simulink model "x12_agv"  (R2025a)
settings: Solver=VariableStepAuto  StartTime=0.0  StopTime=30  RelTol=1e-3
undefined symbols (not defined in the file): Ad, Bd, d_sel, K, kc_pos, kc_vel, p, ref_1, ref_10, ref_11, ref_12, ref_2, ref_3, ref_4, ref_5, ref_6, ref_7, ref_8, ref_9, Ts, x0, x0_1, x0_10, x0_11, x0_12, x0_2, x0_3, x0_4, x0_5, x0_6, x0_7, x0_8, x0_9
(part 2 of 2)

== system x12_agv/agv_init ==
  ref_in : Inport
  p_in : Inport  Port=2
  d_sel_in : Inport  Port=3
  Constant : Constant
  DelaySel : MultiPortSwitch  DataPortOrder=Specify indices  DiagnosticForDefault=None  SaturateOnIntegerOverflow=off  InputSameDT=off
  Gain_k : Gain  Gain=K  Multiplication=Matrix(K*u)
  Gain_neg1 : Gain  Gain=-1  Multiplication=Matrix(K*u)
  Produc_lt : Product
  Product_g : Product
  Relational Operator : RelationalOperator  OutDataTypeStr=boolean  RndMeth=Simplest  InputSameDT=off
  Sum-e : Sum  Inputs=|+-
  plant : DiscreteStateSpace  A=Ad  B=Bd  C=eye(4)  D=zeros(4,2)  InitialCondition=x0  SampleTime=Ts
  sum2 : Sum  Inputs=|++
  sum3 : Sum  Inputs=|++
  ud_u1 : UnitDelay  InitialCondition=[0;0]  SampleTime=Ts  HasFrameUpgradeWarning=on
  ud_u2 : UnitDelay  InitialCondition=[0;0]  SampleTime=Ts  HasFrameUpgradeWarning=on
  ud_u3 : UnitDelay  InitialCondition=[0;0]  SampleTime=Ts  HasFrameUpgradeWarning=on
  ud_ua_prev : UnitDelay  InitialCondition=[0;0]  SampleTime=Ts  HasFrameUpgradeWarning=on
  uniformrandom : UniformRandomNumber  Minimum=0  SampleTime=Ts
  x_out : Outport
  ua_out : Outport  Port=2
  gamma_out : Outport  Port=3
  wires:
  ud_u1/1 -> ud_u2/1, DelaySel/2
  Relational Operator/1 -> gamma_out/1, Product_g/2, Gain_neg1/1
  ud_u3/1 -> DelaySel/4
  plant/1 -> Sum-e/1, x_out/1
  Produc_lt/1 -> sum3/2
  sum2/1 -> Produc_lt/1
  ud_ua_prev/1 -> Produc_lt/2
  Constant/1 -> sum2/2
  Gain_neg1/1 -> sum2/1
  DelaySel/1 -> Product_g/1
  Product_g/1 -> sum3/1
  Gain_k/1 -> ud_u1/1
  ud_u2/1 -> ud_u3/1, DelaySel/3
  Sum-e/1 -> Gain_k/1
  sum3/1 -> ud_ua_prev/1, plant/1, ua_out/1
  uniformrandom/1 -> Relational Operator/1
  ref_in/1 -> Sum-e/2
  p_in/1 -> Relational Operator/2
  d_sel_in/1 -> DelaySel/1

== matlab function x12_agv/Ucoop_8/MATLAB Function ==
  data: xi input; u_coop output; xj1 input; xj2 input; xj3 input; kc_pos input; kc_vel input; u_rep output
function [u_coop, u_rep] = fcn(xi, xj1, xj2, xj3, kc_pos, kc_vel)
% xi, xj1, xj2, xj3: [4x1] = [px; py; vx; vy]

% ----- fixed repulsion params -----
d_safe = 0.45;
k_rep  = 2.4;

% ----- cooperative term (2-neighbor) -----
pi  = xi(1:2);
vi  = xi(3:4);

pj1 = xj1(1:2); vj1 = xj1(3:4);
pj2 = xj2(1:2); vj2 = xj2(3:4);
pj3 = xj3(1:2); % repulsion-only neighbor

e_pos = (pi - pj1) + (pi - pj2);
e_vel = (vi - vj1) + (vi - vj2);

u_coop_base = -kc_pos * e_pos - kc_vel * e_vel;

% ----- repulsion term (3 constraints) -----
eps_d = 1e-6;
u_rep = [0; 0];

% j1
dp = pi - pj1;
d = norm(dp);
if d < d_safe
    u_rep = u_rep + k_rep * (d_safe - d) * (dp / (d + eps_d));
end

% j2
dp = pi - pj2;
d = norm(dp);
if d < d_safe
    u_rep = u_rep + k_rep * (d_safe - d) * (dp / (d + eps_d));
end

% j3
dp = pi - pj3;
d = norm(dp);
if d < d_safe
    u_rep = u_rep + k_rep * (d_safe - d) * (dp / (d + eps_d));
end

% output-1 keeps original channel name u_coop, now includes repulsion
u_coop = u_coop_base + u_rep;
end

== matlab function x12_agv/Ucoop_9/MATLAB Function ==
  data: xi input; u_coop output; xj1 input; xj2 input; xj3 input; kc_pos input; kc_vel input; u_rep output
function [u_coop, u_rep] = fcn(xi, xj1, xj2, xj3, kc_pos, kc_vel)
% xi, xj1, xj2, xj3: [4x1] = [px; py; vx; vy]

% ----- fixed repulsion params -----
d_safe = 0.45;
k_rep  = 2.4;

% ----- cooperative term (2-neighbor) -----
pi  = xi(1:2);
vi  = xi(3:4);

pj1 = xj1(1:2); vj1 = xj1(3:4);
pj2 = xj2(1:2); vj2 = xj2(3:4);
pj3 = xj3(1:2); % repulsion-only neighbor

e_pos = (pi - pj1) + (pi - pj2);
e_vel = (vi - vj1) + (vi - vj2);

u_coop_base = -kc_pos * e_pos - kc_vel * e_vel;

% ----- repulsion term (3 constraints) -----
eps_d = 1e-6;
u_rep = [0; 0];

% j1
dp = pi - pj1;
d = norm(dp);
if d < d_safe
    u_rep = u_rep + k_rep * (d_safe - d) * (dp / (d + eps_d));
end

% j2
dp = pi - pj2;
d = norm(dp);
if d < d_safe
    u_rep = u_rep + k_rep * (d_safe - d) * (dp / (d + eps_d));
end

% j3
dp = pi - pj3;
d = norm(dp);
if d < d_safe
    u_rep = u_rep + k_rep * (d_safe - d) * (dp / (d + eps_d));
end

% output-1 keeps original channel name u_coop, now includes repulsion
u_coop = u_coop_base + u_rep;
end

== matlab function x12_agv/Ucoop_10/MATLAB Function ==
  data: xi input; u_coop output; xj1 input; xj2 input; xj3 input; kc_pos input; kc_vel input; u_rep output
function [u_coop, u_rep] = fcn(xi, xj1, xj2, xj3, kc_pos, kc_vel)
% xi, xj1, xj2, xj3: [4x1] = [px; py; vx; vy]

% ----- fixed repulsion params -----
d_safe = 0.45;
k_rep  = 2.4;

% ----- cooperative term (2-neighbor) -----
pi  = xi(1:2);
vi  = xi(3:4);

pj1 = xj1(1:2); vj1 = xj1(3:4);
pj2 = xj2(1:2); vj2 = xj2(3:4);
pj3 = xj3(1:2); % repulsion-only neighbor

e_pos = (pi - pj1) + (pi - pj2);
e_vel = (vi - vj1) + (vi - vj2);

u_coop_base = -kc_pos * e_pos - kc_vel * e_vel;

% ----- repulsion term (3 constraints) -----
eps_d = 1e-6;
u_rep = [0; 0];

% j1
dp = pi - pj1;
d = norm(dp);
if d < d_safe
    u_rep = u_rep + k_rep * (d_safe - d) * (dp / (d + eps_d));
end

% j2
dp = pi - pj2;
d = norm(dp);
if d < d_safe
    u_rep = u_rep + k_rep * (d_safe - d) * (dp / (d + eps_d));
end

% j3
dp = pi - pj3;
d = norm(dp);
if d < d_safe
    u_rep = u_rep + k_rep * (d_safe - d) * (dp / (d + eps_d));
end

% output-1 keeps original channel name u_coop, now includes repulsion
u_coop = u_coop_base + u_rep;
end

== matlab function x12_agv/Ucoop_11/MATLAB Function ==
  data: xi input; u_coop output; xj1 input; xj2 input; xj3 input; kc_pos input; kc_vel input; u_rep output
function [u_coop, u_rep] = fcn(xi, xj1, xj2, xj3, kc_pos, kc_vel)
% xi, xj1, xj2, xj3: [4x1] = [px; py; vx; vy]

% ----- fixed repulsion params -----
d_safe = 0.45;
k_rep  = 2.4;

% ----- cooperative term (2-neighbor) -----
pi  = xi(1:2);
vi  = xi(3:4);

pj1 = xj1(1:2); vj1 = xj1(3:4);
pj2 = xj2(1:2); vj2 = xj2(3:4);
pj3 = xj3(1:2); % repulsion-only neighbor

e_pos = (pi - pj1) + (pi - pj2);
e_vel = (vi - vj1) + (vi - vj2);

u_coop_base = -kc_pos * e_pos - kc_vel * e_vel;

% ----- repulsion term (3 constraints) -----
eps_d = 1e-6;
u_rep = [0; 0];

% j1
dp = pi - pj1;
d = norm(dp);
if d < d_safe
    u_rep = u_rep + k_rep * (d_safe - d) * (dp / (d + eps_d));
end

% j2
dp = pi - pj2;
d = norm(dp);
if d < d_safe
    u_rep = u_rep + k_rep * (d_safe - d) * (dp / (d + eps_d));
end

% j3
dp = pi - pj3;
d = norm(dp);
if d < d_safe
    u_rep = u_rep + k_rep * (d_safe - d) * (dp / (d + eps_d));
end

% output-1 keeps original channel name u_coop, now includes repulsion
u_coop = u_coop_base + u_rep;
end

== matlab function x12_agv/Ucoop_3/MATLAB Function ==
  data: xi input; u_coop output; xj1 input; xj2 input; xj3 input; kc_pos input; kc_vel input; u_rep output
function [u_coop, u_rep] = fcn(xi, xj1, xj2, xj3, kc_pos, kc_vel)
% xi, xj1, xj2, xj3: [4x1] = [px; py; vx; vy]

% ----- fixed repulsion params -----
d_safe = 0.45;
k_rep  = 2.4;

% ----- cooperative term (2-neighbor) -----
pi  = xi(1:2);
vi  = xi(3:4);

pj1 = xj1(1:2); vj1 = xj1(3:4);
pj2 = xj2(1:2); vj2 = xj2(3:4);
pj3 = xj3(1:2); % repulsion-only neighbor

e_pos = (pi - pj1) + (pi - pj2);
e_vel = (vi - vj1) + (vi - vj2);

u_coop_base = -kc_pos * e_pos - kc_vel * e_vel;

% ----- repulsion term (3 constraints) -----
eps_d = 1e-6;
u_rep = [0; 0];

% j1
dp = pi - pj1;
d = norm(dp);
if d < d_safe
    u_rep = u_rep + k_rep * (d_safe - d) * (dp / (d + eps_d));
end

% j2
dp = pi - pj2;
d = norm(dp);
if d < d_safe
    u_rep = u_rep + k_rep * (d_safe - d) * (dp / (d + eps_d));
end

% j3
dp = pi - pj3;
d = norm(dp);
if d < d_safe
    u_rep = u_rep + k_rep * (d_safe - d) * (dp / (d + eps_d));
end

% output-1 keeps original channel name u_coop, now includes repulsion
u_coop = u_coop_base + u_rep;
end

== matlab function x12_agv/Ucoop_12/MATLAB Function ==
  data: xi input; u_coop output; xj1 input; xj2 input; xj3 input; kc_pos input; kc_vel input; u_rep output
function [u_coop, u_rep] = fcn(xi, xj1, xj2, xj3, kc_pos, kc_vel)
% xi, xj1, xj2, xj3: [4x1] = [px; py; vx; vy]

% ----- fixed repulsion params -----
d_safe = 0.45;
k_rep  = 2.4;

% ----- cooperative term (2-neighbor) -----
pi  = xi(1:2);
vi  = xi(3:4);

pj1 = xj1(1:2); vj1 = xj1(3:4);
pj2 = xj2(1:2); vj2 = xj2(3:4);
pj3 = xj3(1:2); % repulsion-only neighbor

e_pos = (pi - pj1) + (pi - pj2);
e_vel = (vi - vj1) + (vi - vj2);

u_coop_base = -kc_pos * e_pos - kc_vel * e_vel;

% ----- repulsion term (3 constraints) -----
eps_d = 1e-6;
u_rep = [0; 0];

% j1
dp = pi - pj1;
d = norm(dp);
if d < d_safe
    u_rep = u_rep + k_rep * (d_safe - d) * (dp / (d + eps_d));
end

% j2
dp = pi - pj2;
d = norm(dp);
if d < d_safe
    u_rep = u_rep + k_rep * (d_safe - d) * (dp / (d + eps_d));
end

% j3
dp = pi - pj3;
d = norm(dp);
if d < d_safe
    u_rep = u_rep + k_rep * (d_safe - d) * (dp / (d + eps_d));
end

% output-1 keeps original channel name u_coop, now includes repulsion
u_coop = u_coop_base + u_rep;
end

== matlab function x12_agv/Ucoop_1/MATLAB Function ==
  data: xi input; u_coop output; xj1 input; xj2 input; xj3 input; kc_pos input; kc_vel input; u_rep output
function [u_coop, u_rep] = fcn(xi, xj1, xj2, xj3, kc_pos, kc_vel)
% xi, xj1, xj2, xj3: [4x1] = [px; py; vx; vy]

% ----- fixed repulsion params -----
d_safe = 0.45;
k_rep  = 2.4;

% ----- cooperative term (2-neighbor) -----
pi  = xi(1:2);
vi  = xi(3:4);

pj1 = xj1(1:2); vj1 = xj1(3:4);
pj2 = xj2(1:2); vj2 = xj2(3:4);
pj3 = xj3(1:2); % repulsion-only neighbor

e_pos = (pi - pj1) + (pi - pj2);
e_vel = (vi - vj1) + (vi - vj2);

u_coop_base = -kc_pos * e_pos - kc_vel * e_vel;

% ----- repulsion term (3 constraints) -----
eps_d = 1e-6;
u_rep = [0; 0];

% j1
dp = pi - pj1;
d = norm(dp);
if d < d_safe
    u_rep = u_rep + k_rep * (d_safe - d) * (dp / (d + eps_d));
end

% j2
dp = pi - pj2;
d = norm(dp);
if d < d_safe
    u_rep = u_rep + k_rep * (d_safe - d) * (dp / (d + eps_d));
end

% j3
dp = pi - pj3;
d = norm(dp);
if d < d_safe
    u_rep = u_rep + k_rep * (d_safe - d) * (dp / (d + eps_d));
end

% output-1 keeps original channel name u_coop, now includes repulsion
u_coop = u_coop_base + u_rep;
end

== matlab function x12_agv/Ucoop_2/MATLAB Function ==
  data: xi input; u_coop output; xj1 input; xj2 input; xj3 input; kc_pos input; kc_vel input; u_rep output
function [u_coop, u_rep] = fcn(xi, xj1, xj2, xj3, kc_pos, kc_vel)
% xi, xj1, xj2, xj3: [4x1] = [px; py; vx; vy]

% ----- fixed repulsion params -----
d_safe = 0.45;
k_rep  = 2.4;

% ----- cooperative term (2-neighbor) -----
pi  = xi(1:2);
vi  = xi(3:4);

pj1 = xj1(1:2); vj1 = xj1(3:4);
pj2 = xj2(1:2); vj2 = xj2(3:4);
pj3 = xj3(1:2); % repulsion-only neighbor

e_pos = (pi - pj1) + (pi - pj2);
e_vel = (vi - vj1) + (vi - vj2);

u_coop_base = -kc_pos * e_pos - kc_vel * e_vel;

% ----- repulsion term (3 constraints) -----
eps_d = 1e-6;
u_rep = [0; 0];

% j1
dp = pi - pj1;
d = norm(dp);
if d < d_safe
    u_rep = u_rep + k_rep * (d_safe - d) * (dp / (d + eps_d));
end

% j2
dp = pi - pj2;
d = norm(dp);
if d < d_safe
    u_rep = u_rep + k_rep * (d_safe - d) * (dp / (d + eps_d));
end

% j3
dp = pi - pj3;
d = norm(dp);
if d < d_safe
    u_rep = u_rep + k_rep * (d_safe - d) * (dp / (d + eps_d));
end

% output-1 keeps original channel name u_coop, now includes repulsion
u_coop = u_coop_base + u_rep;
end

== matlab function x12_agv/Ucoop_4/MATLAB Function ==
  data: xi input; u_coop output; xj1 input; xj2 input; xj3 input; kc_pos input; kc_vel input; u_rep output
function [u_coop, u_rep] = fcn(xi, xj1, xj2, xj3, kc_pos, kc_vel)
% xi, xj1, xj2, xj3: [4x1] = [px; py; vx; vy]

% ----- fixed repulsion params -----
d_safe = 0.45;
k_rep  = 2.4;

% ----- cooperative term (2-neighbor) -----
pi  = xi(1:2);
vi  = xi(3:4);

pj1 = xj1(1:2); vj1 = xj1(3:4);
pj2 = xj2(1:2); vj2 = xj2(3:4);
pj3 = xj3(1:2); % repulsion-only neighbor

e_pos = (pi - pj1) + (pi - pj2);
e_vel = (vi - vj1) + (vi - vj2);

u_coop_base = -kc_pos * e_pos - kc_vel * e_vel;

% ----- repulsion term (3 constraints) -----
eps_d = 1e-6;
u_rep = [0; 0];

% j1
dp = pi - pj1;
d = norm(dp);
if d < d_safe
    u_rep = u_rep + k_rep * (d_safe - d) * (dp / (d + eps_d));
end

% j2
dp = pi - pj2;
d = norm(dp);
if d < d_safe
    u_rep = u_rep + k_rep * (d_safe - d) * (dp / (d + eps_d));
end

% j3
dp = pi - pj3;
d = norm(dp);
if d < d_safe
    u_rep = u_rep + k_rep * (d_safe - d) * (dp / (d + eps_d));
end

% output-1 keeps original channel name u_coop, now includes repulsion
u_coop = u_coop_base + u_rep;
end

== matlab function x12_agv/Ucoop_5/MATLAB Function ==
  data: xi input; u_coop output; xj1 input; xj2 input; xj3 input; kc_pos input; kc_vel input; u_rep output
function [u_coop, u_rep] = fcn(xi, xj1, xj2, xj3, kc_pos, kc_vel)
% xi, xj1, xj2, xj3: [4x1] = [px; py; vx; vy]

% ----- fixed repulsion params -----
d_safe = 0.45;
k_rep  = 2.4;

% ----- cooperative term (2-neighbor) -----
pi  = xi(1:2);
vi  = xi(3:4);

pj1 = xj1(1:2); vj1 = xj1(3:4);
pj2 = xj2(1:2); vj2 = xj2(3:4);
pj3 = xj3(1:2); % repulsion-only neighbor

e_pos = (pi - pj1) + (pi - pj2);
e_vel = (vi - vj1) + (vi - vj2);

u_coop_base = -kc_pos * e_pos - kc_vel * e_vel;

% ----- repulsion term (3 constraints) -----
eps_d = 1e-6;
u_rep = [0; 0];

% j1
dp = pi - pj1;
d = norm(dp);
if d < d_safe
    u_rep = u_rep + k_rep * (d_safe - d) * (dp / (d + eps_d));
end

% j2
dp = pi - pj2;
d = norm(dp);
if d < d_safe
    u_rep = u_rep + k_rep * (d_safe - d) * (dp / (d + eps_d));
end

% j3
dp = pi - pj3;
d = norm(dp);
if d < d_safe
    u_rep = u_rep + k_rep * (d_safe - d) * (dp / (d + eps_d));
end

% output-1 keeps original channel name u_coop, now includes repulsion
u_coop = u_coop_base + u_rep;
end

== matlab function x12_agv/Ucoop_6/MATLAB Function ==
  data: xi input; u_coop output; xj1 input; xj2 input; xj3 input; kc_pos input; kc_vel input; u_rep output
function [u_coop, u_rep] = fcn(xi, xj1, xj2, xj3, kc_pos, kc_vel)
% xi, xj1, xj2, xj3: [4x1] = [px; py; vx; vy]

% ----- fixed repulsion params -----
d_safe = 0.45;
k_rep  = 2.4;

% ----- cooperative term (2-neighbor) -----
pi  = xi(1:2);
vi  = xi(3:4);

pj1 = xj1(1:2); vj1 = xj1(3:4);
pj2 = xj2(1:2); vj2 = xj2(3:4);
pj3 = xj3(1:2); % repulsion-only neighbor

e_pos = (pi - pj1) + (pi - pj2);
e_vel = (vi - vj1) + (vi - vj2);

u_coop_base = -kc_pos * e_pos - kc_vel * e_vel;

% ----- repulsion term (3 constraints) -----
eps_d = 1e-6;
u_rep = [0; 0];

% j1
dp = pi - pj1;
d = norm(dp);
if d < d_safe
    u_rep = u_rep + k_rep * (d_safe - d) * (dp / (d + eps_d));
end

% j2
dp = pi - pj2;
d = norm(dp);
if d < d_safe
    u_rep = u_rep + k_rep * (d_safe - d) * (dp / (d + eps_d));
end

% j3
dp = pi - pj3;
d = norm(dp);
if d < d_safe
    u_rep = u_rep + k_rep * (d_safe - d) * (dp / (d + eps_d));
end

% output-1 keeps original channel name u_coop, now includes repulsion
u_coop = u_coop_base + u_rep;
end

== matlab function x12_agv/Ucoop_7/MATLAB Function ==
  data: xi input; u_coop output; xj1 input; xj2 input; xj3 input; kc_pos input; kc_vel input; u_rep output
function [u_coop, u_rep] = fcn(xi, xj1, xj2, xj3, kc_pos, kc_vel)
% xi, xj1, xj2, xj3: [4x1] = [px; py; vx; vy]

% ----- fixed repulsion params -----
d_safe = 0.45;
k_rep  = 2.4;

% ----- cooperative term (2-neighbor) -----
pi  = xi(1:2);
vi  = xi(3:4);

pj1 = xj1(1:2); vj1 = xj1(3:4);
pj2 = xj2(1:2); vj2 = xj2(3:4);
pj3 = xj3(1:2); % repulsion-only neighbor

e_pos = (pi - pj1) + (pi - pj2);
e_vel = (vi - vj1) + (vi - vj2);

u_coop_base = -kc_pos * e_pos - kc_vel * e_vel;

% ----- repulsion term (3 constraints) -----
eps_d = 1e-6;
u_rep = [0; 0];

% j1
dp = pi - pj1;
d = norm(dp);
if d < d_safe
    u_rep = u_rep + k_rep * (d_safe - d) * (dp / (d + eps_d));
end

% j2
dp = pi - pj2;
d = norm(dp);
if d < d_safe
    u_rep = u_rep + k_rep * (d_safe - d) * (dp / (d + eps_d));
end

% j3
dp = pi - pj3;
d = norm(dp);
if d < d_safe
    u_rep = u_rep + k_rep * (d_safe - d) * (dp / (d + eps_d));
end

% output-1 keeps original channel name u_coop, now includes repulsion
u_coop = u_coop_base + u_rep;
end
